simulink library "VelocityController_v0_CL"  (R2020a)
settings: Solver=VariableStepAuto  StartTime=0.0  StopTime=10.0  RelTol=1e-3
undefined symbols (not defined in the file): ICE, Int, sig_info, UNCC, VEH
libraries: Thesis_Sublibraries x5, MPC_51_v0_CL x1
settings Model: Creator=John Jr  LastModifiedBy=John Jr

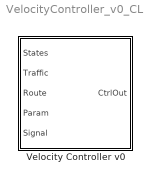
== system VelocityController_v0_CL ==
  Velocity Controller v0 : Subsystem  TreatAsAtomicUnit=on
      mask Display:
      | patch([0 1 1 0], [0 0 1 1],[1 .8 1])
      | 
      | port_label('input',1,'\fontname{Cambria Math}States','texmode','on')
      | port_label('input',2,'\fontname{Cambria Math}Traffic','texmode','on')
      | port_label('input',3,'\fontname{Cambria Math}Route','texmode','on')
      | port_label('input',4,'\fontname{Cambria Math}Param','texmode','on')
      | port_label('input',5,'\fontname{Cambria Math}Signal','texmode','on')
      | 
      | port_label('output',1,'\fontname{Cambria Math}CtrlOut','texmode','on')

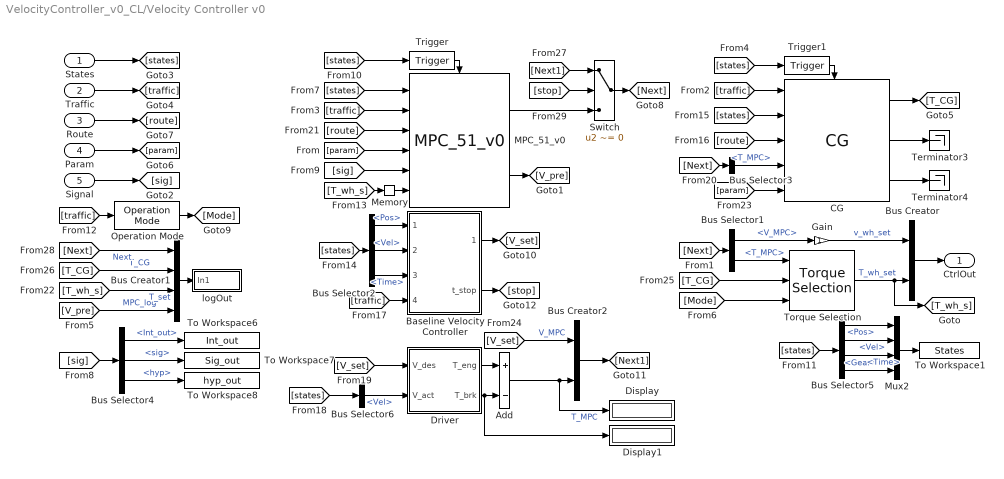
== system VelocityController_v0_CL/Velocity Controller v0 ==
  States : Inport
  Traffic : Inport  Port=2
  Route : Inport  Port=3
  Param : Inport  Port=4
  Signal : Inport  Port=5
  Add : Sum  Inputs=+-
  Baseline Velocity Controller : Subsystem
      mask Display:
      | patch([0 1 1 0], [0 0 1 1],[.8 1 1])
      | 
      | port_label('input',1,'Position','texmode','on')
      | port_label('input',2,'Velocity','texmode','on')
      | port_label('input',4,'Traffic','texmode','on')
      | port_label('input',3,'Time','texmode','on')
      | 
      | port_label('output',1,'V_{set}','texmode','on')
      | port_label('output',2,'t_{stop}','texmode','on')
  Bus Creator : BusCreator  Inputs=2
  Bus Creator1 : BusCreator  Inputs=4
  Bus Creator2 : BusCreator  Inputs=2
  Bus Selector1 : BusSelector  OutputSignals=V_MPC,T_MPC
  Bus Selector2 : BusSelector  OutputSignals=Pos,Vel,Time
  Bus Selector3 : BusSelector  OutputSignals=T_MPC
  Bus Selector4 : BusSelector  OutputSignals=Int_out,sig,hyp
  Bus Selector5 : BusSelector  OutputSignals=Pos,Vel,Time,Gear
  Bus Selector6 : BusSelector  OutputSignals=Vel
  CG : Thesis_Sublibraries/CG  SystemSampleTime=-1  Latency=0  AutoFrameSizeCalculation=off
  Display : Display
  Display1 : Display
  Driver : Subsystem
  Gain : Gain
  MPC_51_v0 : MPC_51_v0_CL/MPC_51_v0  SystemSampleTime=-1  Latency=0  AutoFrameSizeCalculation=off
  Memory : Memory  InitialCondition=11
  Mux2 : Mux
  Operation Mode : Thesis_Sublibraries/Operation Mode  ds_max=200
  Switch : Switch  Criteria=u2 ~= 0  ZeroCross=off
  Terminator3 : Terminator
  Terminator4 : Terminator
  To Workspace1 : ToWorkspace  VariableName=States  SampleTime=-1
  To Workspace6 : ToWorkspace  VariableName=Int_out  SampleTime=-1
  To Workspace7 : ToWorkspace  VariableName=Sig_out  SampleTime=-1
  To Workspace8 : ToWorkspace  VariableName=hyp_out  SampleTime=-1
  Torque Selection : Thesis_Sublibraries/Torque Selection  SystemSampleTime=-1  Latency=0  AutoFrameSizeCalculation=off
  Trigger : Thesis_Sublibraries/Trigger  f=1
  Trigger1 : Thesis_Sublibraries/Trigger  f=2.5
  logOut : Subsystem
      mask Display:
      | patch([0 1 1 0], [0 0 1 1],[.8 1 .8])
      | 
      | port_label('input',1,'Log Out')
  CtrlOut : Outport  VectorParamsAs1DForOutWhenUnconnected=off
  wires:
  Traffic/1 -> [traffic]
  Route/1 -> [route]
  States/1 -> [states]
  [states] -> Trigger/1
  Trigger/1 -> MPC_51_v0/Trigger
  [route] -> MPC_51_v0/3
  [param] -> MPC_51_v0/4
  [traffic] -> MPC_51_v0/2
  [states] -> MPC_51_v0/1
  Param/1 -> [param]
  Gain/1 -> Bus Creator/1  "v_wh_set"
  Bus Selector1/1 -> Gain/1  "<V_MPC>"
  Bus Selector1/2 -> Torque Selection/1  "<T_MPC>"
  [Mode] -> Torque Selection/3
  [Next] -> Bus Selector1/1
  Torque Selection/1 -> [T_wh_s], Bus Creator/2  "T_wh_set"
  [T_CG] -> Torque Selection/2
  Bus Creator/1 -> CtrlOut/1
  CG/3 -> Terminator4/1
  [Next] -> Bus Selector3/1
  [param] -> CG/5
  CG/1 -> [T_CG]
  Bus Selector3/1 -> CG/4  "<T_MPC>"
  [route] -> CG/3
  Trigger1/1 -> CG/Trigger
  [states] -> Trigger1/1
  CG/2 -> Terminator3/1
  [states] -> CG/2
  [traffic] -> CG/1
  [V_pre] -> Bus Creator1/4  "MPC_log"
  [T_CG] -> Bus Creator1/2  "T_CG"
  [T_wh_s] -> Bus Creator1/3  "T_set"
  [Next] -> Bus Creator1/1  "Next"
  Bus Creator1/1 -> logOut/1(In1)
  Signal/1 -> [sig]
  MPC_51_v0/2 -> [V_pre]
  [sig] -> MPC_51_v0/5
  Memory/1 -> MPC_51_v0/6
  [T_wh_s] -> Memory/1
  [sig] -> Bus Selector4/1
  Bus Selector4/1 -> To Workspace6/1  "<Int_out>"
  Bus Selector4/3 -> To Workspace8/1  "<hyp>"
  Bus Selector4/2 -> To Workspace7/1  "<sig>"
  Bus Selector5/4 -> Mux2/4  "<Gear>"
  Bus Selector5/1 -> Mux2/1  "<Pos>"
  Mux2/1 -> To Workspace1/1
  Bus Selector5/2 -> Mux2/2  "<Vel>"
  Bus Selector5/3 -> Mux2/3  "<Time>"
  [states] -> Bus Selector5/1
  [traffic] -> Operation Mode/1
  Operation Mode/1 -> [Mode]
  [states] -> Bus Selector2/1
  Bus Selector2/3 -> Baseline Velocity Controller/3(Time [s])  "<Time>"
  Bus Selector2/2 -> Baseline Velocity Controller/2(Velocity [m/s])  "<Vel>"
  Bus Selector2/1 -> Baseline Velocity Controller/1(Position [m])  "<Pos>"
  [traffic] -> Baseline Velocity Controller/4(Traffic Info)
  Driver/2(T_brk) -> Display1/1, Add/2
  Bus Selector6/1 -> Driver/2(V_act)  "<Vel>"
  Driver/1(T_eng) -> Add/1
  [V_set] -> Driver/1(V_des)
  Baseline Velocity Controller/1(Target Velocity [m/s]) -> [V_set]
  Baseline Velocity Controller/2(t_stop) -> [stop]
  Bus Creator2/1 -> [Next1]
  Switch/1 -> [Next]
  [stop] -> Switch/2
  MPC_51_v0/1 -> Switch/3
  [Next1] -> Switch/1
  [V_set] -> Bus Creator2/1  "V_MPC"
  Add/1 -> Display/1, Bus Creator2/2  "T_MPC"
  [states] -> Bus Selector6/1

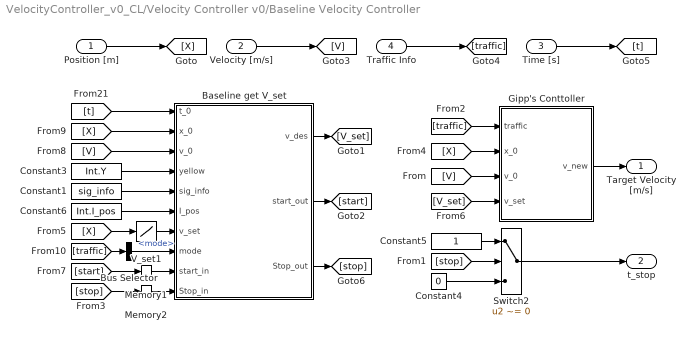
== system VelocityController_v0_CL/Velocity Controller v0/Baseline Velocity Controller ==
  Position [m] : Inport
  Velocity [m/s] : Inport  Port=2
  Time [s] : Inport  Port=3
  Traffic Info : Inport  Port=4
  Baseline get V_set : MATLAB Function  TreatAsAtomicUnit=on
  Bus Selector : BusSelector  OutputSignals=mode
  Constant1 : Constant  Value=sig_info
  Constant3 : Constant  Value=Int.Y
  Constant4 : Constant  Value=0
  Constant5 : Constant
  Constant6 : Constant  Value=Int.I_pos
  Gipp's Conttoller : MATLAB Function  TreatAsAtomicUnit=on
  Memory1 : Memory  InitialCondition=[0 0]
  Memory2 : Memory
  Switch2 : Switch  Criteria=u2 ~= 0
  V_set1 : Lookup_n-D  NumberOfTableDimensions=1  BreakpointsForDimension1=UNCC.X_vec  Table=UNCC.V_lim  InterpMethod=Flat  ExtrapMethod=Clip  InputSameDT=on
  Target Velocity [m/s] : Outport  VectorParamsAs1DForOutWhenUnconnected=off
  t_stop : Outport  Port=2  VectorParamsAs1DForOutWhenUnconnected=off
  wires:
  Gipp's Conttoller/1(v_new) -> Target Velocity [m/s]/1
  [start] -> Memory1/1
  [stop] -> Memory2/1
  Memory2/1 -> Baseline get V_set/10(Stop_in)
  Memory1/1 -> Baseline get V_set/9(start_in)
  [stop] -> Switch2/2
  Baseline get V_set/3(Stop_out) -> [stop]
  Baseline get V_set/2(start_out) -> [start]
  Switch2/1 -> t_stop/1
  Constant5/1 -> Switch2/1
  Constant4/1 -> Switch2/3
  [V_set] -> Gipp's Conttoller/4(v_set)
  [V] -> Baseline get V_set/3(v_0)
  Baseline get V_set/1(v_des) -> [V_set]
  Constant3/1 -> Baseline get V_set/4(yellow)
  [X] -> Baseline get V_set/2(x_0)
  Constant1/1 -> Baseline get V_set/5(sig_info)
  V_set1/1 -> Baseline get V_set/7(v_set)
  [t] -> Baseline get V_set/1(t_0)
  Constant6/1 -> Baseline get V_set/6(I_pos)
  [X] -> V_set1/1
  Time [s]/1 -> [t]
  [V] -> Gipp's Conttoller/3(v_0)
  Velocity [m/s]/1 -> [V]
  Traffic Info/1 -> [traffic]
  [X] -> Gipp's Conttoller/2(x_0)
  [traffic] -> Gipp's Conttoller/1(traffic)
  Position [m]/1 -> [X]
  [traffic] -> Bus Selector/1
  Bus Selector/1 -> Baseline get V_set/8(mode)  "<mode>"

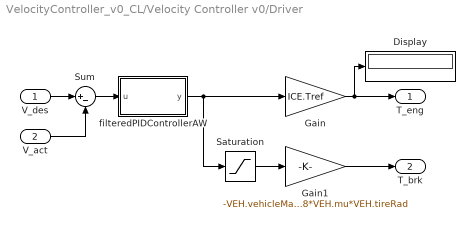
== system VelocityController_v0_CL/Velocity Controller v0/Driver ==
  V_des : Inport
  V_act : Inport  Port=2
  Display : Display
  Gain : Gain  Gain=ICE.Tref
  Gain1 : Gain  Gain=-VEH.vehicleMass*9.8*VEH.mu*VEH.tireRad
  Saturation : Saturate  UpperLimit=0  LowerLimit=-1
  Sum : Sum  Inputs=|+-
  filteredPIDControllerAW : Subsystem  mask{kp=5, ki=1, kd=0, tau=.01, cmax=1, cmin=-1}
      mask prompts: kp "Proportional Gain, kp"; ki "Integral Gain, ki"; kd "Derivative Gain, kd"; tau "Time Constant, s"; cmax "Control Upper Limit"; cmin "Control Lower Limit"
  T_eng : Outport  VectorParamsAs1DForOutWhenUnconnected=off
  T_brk : Outport  Port=2  VectorParamsAs1DForOutWhenUnconnected=off
  wires:
  Sum/1 -> filteredPIDControllerAW/1(u)
  Saturation/1 -> Gain1/1
  V_des/1 -> Sum/1
  V_act/1 -> Sum/2
  Gain1/1 -> T_brk/1
  filteredPIDControllerAW/1(y) -> Saturation/1, Gain/1
  Gain/1 -> Display/1, T_eng/1

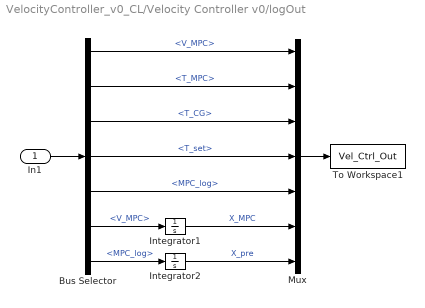
== system VelocityController_v0_CL/Velocity Controller v0/logOut ==
  In1 : Inport
  Bus Selector : BusSelector  OutputSignals=Next.V_MPC,Next.T_MPC,T_CG,T_set,MPC_log,Next.V_MPC,MPC_log
  Integrator1 : Integrator
  Integrator2 : Integrator
  Mux : Mux  Inputs=7
  To Workspace1 : ToWorkspace  VariableName=Vel_Ctrl_Out  SaveFormat=Structure With Time  SampleTime=-1
  wires:
  Bus Selector/4 -> Mux/4  "<T_set>"
  Bus Selector/3 -> Mux/3  "<T_CG>"
  Bus Selector/2 -> Mux/2  "<T_MPC>"
  Bus Selector/1 -> Mux/1  "<V_MPC>"
  Mux/1 -> To Workspace1/1
  In1/1 -> Bus Selector/1
  Bus Selector/5 -> Mux/5  "<MPC_log>"
  Bus Selector/6 -> Integrator1/1  "<V_MPC>"
  Bus Selector/7 -> Integrator2/1  "<MPC_log>"
  Integrator1/1 -> Mux/6  "X_MPC"
  Integrator2/1 -> Mux/7  "X_pre"

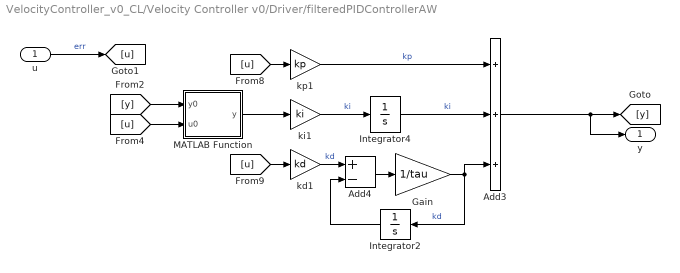
== system VelocityController_v0_CL/Velocity Controller v0/Driver/filteredPIDControllerAW ==
  u : Inport  PortDimensions=1
  Add3 : Sum  Inputs=+++
  Add4 : Sum  Inputs=+-
  Gain : Gain  Gain=1/tau
  Integrator2 : Integrator
  Integrator4 : Integrator
  MATLAB Function : MATLAB Function  TreatAsAtomicUnit=on  mask{cMax=cmax, cMin=cmin}
      mask prompts: cMax "Max control value:"; cMin "Min control value:"
  kd1 : Gain  Gain=kd
  ki1 : Gain  Gain=ki
  kp1 : Gain  Gain=kp
  y : Outport  PortDimensions=1  VectorParamsAs1DForOutWhenUnconnected=off
  wires:
  [u] -> MATLAB Function/2(u0)
  [y] -> MATLAB Function/1(y0)
  u/1 -> [u]  "err"
  kd1/1 -> Add4/1  "kd"
  Integrator2/1 -> Add4/2
  Integrator4/1 -> Add3/2  "ki"
  kp1/1 -> Add3/1  "kp"
  Add4/1 -> Gain/1
  [u] -> kp1/1
  ki1/1 -> Integrator4/1  "ki"
  Gain/1 -> Add3/3, Integrator2/1  "kd"
  [u] -> kd1/1
  MATLAB Function/1(y) -> ki1/1
  Add3/1 -> y/1, [y]

== matlab function VelocityController_v0_CL/Velocity Controller v0/Driver/filteredPIDControllerAW/MATLAB Function ==
  data: y0 input; u0 input; y output; cMax parameter; cMin parameter
function y = fcn(y0, u0, cMax, cMin)

if y0 > cMax
    y1 = cMax; 
elseif y0 < cMin
    y1 = cMin; 
else
    y1 = y0; 
end

sat = y0-y1; 
aw = exp(-1e5*sat^2); 
y = aw*u0;

== matlab function VelocityController_v0_CL/Velocity Controller v0/Baseline Velocity Controller/Baseline get V_set ==
  data: t_0 input; v_des output size=1; start_out output size=[1 2]; x_0 input; v_0 input; yellow input; sig_info input; I_pos input; v_set input; mode input; start_in input size=2; Stop_in input size=1; Stop_out output size=1
function [v_des,start_out,Stop_out] = fcn(t_0,x_0,v_0,yellow,sig_info,I_pos,v_set,mode,start_in,Stop_in)

G = sig_info(:,:,2);                                    %   s - Intersection green phases 
Cs = sig_info(:,:,3);                                   %   s - Cycle start times 
window = 150;                                           %   m - Driver sight range
dt = .01;                                               %   s - Sample time
Idx1 = find(x_0-I_pos < 0,1,'first');                   %   Next upcoming intersection 
if isempty(Idx1)
    dx = 500;
else
    dx = I_pos(Idx1(1))-x_0;                            %   m - Distance to upcoming intersection 
end
if dx >= window
    Int_approach = 0;                                   %   No upcoming intersection 
else
    Int_approach = 1;                                   %   There is an upcoming intersection 
end
if Int_approach == 1
    Idx2 = find(Cs(Idx1(1),:) <= t_0,1,'last');         %   Current cycle # for upcoming intersection
    x_approach = v_0*yellow(Idx1(1));                            %   m - Distance to make yellow
    if t_0 < Cs(Idx1(1),Idx2(1))+G(Idx1(1),Idx2(1))-yellow(Idx1(1))
        light = 0;                                      %   Light is green
    elseif t_0 >= Cs(Idx1(1),Idx2(1))+G(Idx1(1),Idx2(1))-yellow(Idx1(1))...
            && t_0 < Cs(Idx1(1),Idx2(1))+G(Idx1(1),Idx2(1))
        light = 1;                                      %   Light is yellow
    else
        light = 2;                                      %   Light is red
    end
    if light == 0 && Stop_in == 1
        Stop_out = 0;
        start_in = [0 0];
    elseif (light == 1 && dx > x_approach) || light == 2 ...
            || (light == 1 && Stop_in == 1)
        Stop_out = 1;
        start_in = start_in';
    else
        Stop_out = 0;
        start_in = [0 0];
    end
else
    Stop_out = 0;
    start_in = [0 0];
end
if Stop_out == 1 && start_in(1) == 0
    start_in = [x_0,v_0];
end
if Stop_out == 1
    if mode == 1
        x_stop = linspace(start_in(1),I_pos(Idx1(1))-15,100);
    else
        x_stop = linspace(start_in(1),I_pos(Idx1(1))-5,100);
    end
    v_stop = linspace(start_in(2),0,100);
    v_des = interp1(x_stop,v_stop,x_0,'linear',0);
else
    v_des = v_set;
end
start_out = start_in;
end

== matlab function VelocityController_v0_CL/Velocity Controller v0/Baseline Velocity Controller/Gipp's Conttoller ==
  data: traffic input size=6; v_new output; x_0 input; v_0 input; v_set input
function v_new  = fcn(traffic,x_0,v_0,v_set)

tau = 0.75;                 %   s - Driver reaction time
a_n = 2;                    %   m/s^2 - Maximum acceleration
b_n = -2*a_n;               %   m/s^2 - Maximum brake acceleration
b_hat = -2;                 %   m/s^2 - Estimated lead vehicle brake acceleration
t_n = 2;                    %   s - Safe following time

x_lead = traffic(1);        %   m - Lead vehicle poaition
v_lead = traffic(2);        %   m/s - Lead vehicle velocity
s_n = max(v_lead*t_n,5);    %   m - Safe following distance
v_0 = max(v_0,0);

if x_lead-x_0 <= 0          %   Condition to prevent negative radical
    x_lead = x_0;
    v_lead = v_0;
end

if traffic(4) == 0        %   In traffic?
    v_new = v_set;
else
    if (b_n^2*tau^2-b_n*(2*(x_lead-s_n-x_0)-v_0*tau-v_lead^2/b_hat)) > 0
        v_new = min(v_0+2.5*a_n*tau*(1-v_0/v_set)*sqrt(.025+v_0/v_set),...
            b_n*tau+sqrt(b_n^2*tau^2-b_n*(2*(x_lead-s_n-x_0)-v_0*tau-v_lead^2/b_hat)));
    else
        v_new = 0;
    end
    v_new = max(v_new,0);
end
